simulink model "TestHz"  (R2020b)
settings: Solver=FixedStepDiscrete  StartTime=0.0  StopTime=inf  FixedStep=Ts  RelTol=1e-3
values from neighbouring files (symbols this model uses):
  g = 9.81    [equpoint.m]    (also in plotAMS.m; plotAMS2.m)
  J = diag([0.0056 0.0056 0.0104])    [equpoint.m]
  m = 0.7    [equpoint.m]    (also in plotAMS.m = 0.752; plotAMS2.m = 0.752)
  M = ([ 1          1          1         1 ... (first row only)    [allocation.m]    (also in equpoint.m; plotAMS.m; plotAMS2.m)
undefined symbols (not defined in the file or in its folder): B, MY_ATT_P, MY_ATT_P_YAW, MY_POS_P, MY_RATE_P, MY_RATE_P_YAW, MY_SAT_AD, MY_TAU_P_A, MY_TAU_P_A_YAW, MY_TAU_P_P, MY_TAU_P_P_YAW, MY_VEL_P, T00, Tf, Tmotorbar, Ts
libraries: discretizing x10, pixhawk_slib_uORB_RW x6, pixhawk_slib_sensors_actuators x5, pixhawk_slib_misc_utils x1, simulink x1, sharedtransform x1, pid_lib x1
(part 1 of 2)
settings Model: Creator=kcx06  LastModifiedBy=kcx06
settings SolverCC: PositivePriorityOrder=on  AutoInsertRateTranBlk=on
settings DataIOCC: SaveOutput=off  DSMLogging=off  SaveTime=off  ReturnWorkspaceOutputs=off
settings OptimizationCC: DefaultParameterBehavior=Inlined  EnhancedBackFolding=on  PassReuseOutputArgsAs=Individual arguments  ZeroExternalMemoryAtStartup=off  ZeroInternalMemoryAtStartup=off  MaxStackSize=64  OptimizeBlockOrder=speed  DifferentSizesBufferReuse=on  OptimizationCustomize=off  EfficientTunableParamExpr=on
settings DebuggingCC: ParameterTunabilityLossMsg=error
settings HardwareCC: ProdBitPerPointer=32  ProdBitPerSizeT=32  ProdBitPerPtrDiffT=32  ProdLargestAtomicInteger=Long  ProdLargestAtomicFloat=Double  ProdWordSize=32  ProdHWDeviceType=ARM Compatible->ARM Cortex
settings SFSimCC: MATLABDynamicMemAlloc=off
settings RTWCC: Description=Embedded Coder  SystemTargetFile=ert.tlc  HardwareBoard=Pixhawk PX4  TLCOptions="-aInlineSetEventsForThisBaseRateFcn=TLC_FALSE -aSuppressMultiTaskScheduler=TLC_FALSE  -aRateBasedStepFcn=0"  TemplateMakefile=ert_default_tmf  GenerateReport=on  CustomSource=px4_simulink_app_params.c  Toolchain=Pixhawk Toolchain  BuildConfiguration=Faster Runs  LaunchReport=on
settings CodeAppCC: ForceParamTrailComments=on  IgnoreCustomStorageClasses=off  OperatorAnnotations=on  SimulinkDataObjDesc=on  SFDataObjDesc=on  InsertBlockDesc=on
settings ERTTargetCC: SupportComplex=off  SupportContinuousTime=on  InlinedParameterPlacement=NonHierarchical  ERTCustomFileTemplate=px4_codertarget_file_process.tlc

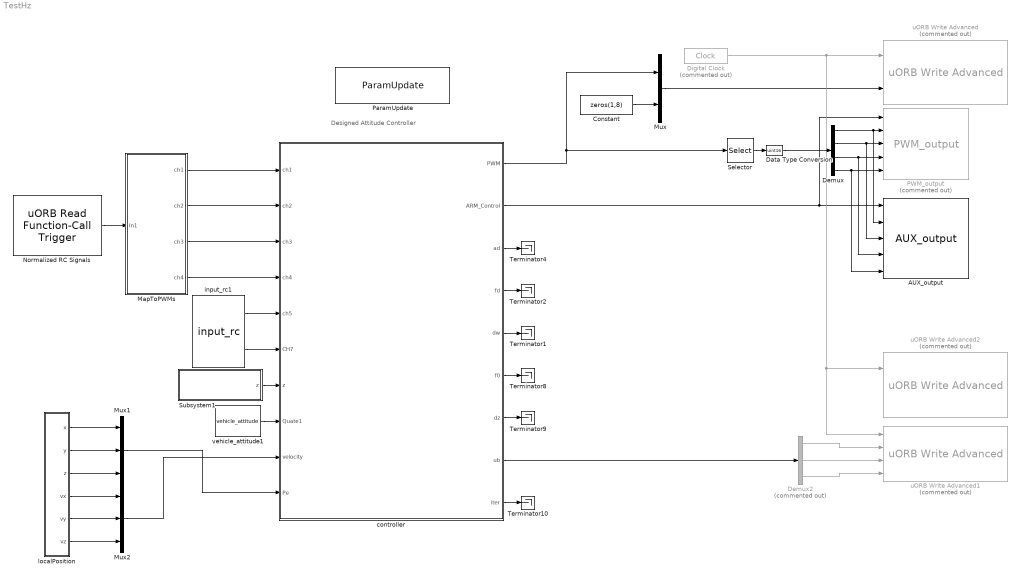
== system TestHz ==
  note: Designed Attitude Controller
  AUX_output : pixhawk_slib_sensors_actuators/AUX_output  Description=|  pwm_rate=400Hz  show_aux1=on  show_aux4=on  show_aux2=on  show_aux5=off  show_aux3=on  show_aux6=off
      | This block allows the user to send the appropriate PWM signals out to the PX4 AUX outputs.  
      | These are usually connected to the ESCs which control the motor speeds. 
      | In order for the flight control to arm (enable) the output from the software side, the ARM Output input must be held high (boolean TRUE).  
      | Only then will the PWM values be sent out the PX4 hardware ports.  
      | This is usually a function of the RC Tx in combination with other flight modes programmed in the Simulink model by the user.  
      | The block has 8 available ports (data type uint16) which can be selectively chosen.  
      | These correspond to the 6 PWM (optional on 5/6) output ports on the px4fmu hardware. 
      | 
      | You *must* ensure that the line: “fmu mode_pwm” appears in your rc.txt file or manually run this from a Nuttx terminal *before* you start the px4_simulink_app module.  
      | Also – note: the FMU only has to be ARMED for the AUX pins to work – the Hardware safety switch is only for the IO.  
      | The switch’s blink code tells you what is armed.  You have to ARM both the Hardware switch and Software block in order to get the PWM output to work, but only the Software block for the AUX outputs.
      settings: SourceProductName=Pixhawk Target Blocks
  Constant : Constant  Value=zeros(1,8)  OutDataTypeStr=single
  Data Type Conversion : DataTypeConversion  OutDataTypeStr=uint16
  Demux : Demux
  Demux2 : Demux  Commented=on  Outputs=3
  Digital Clock : DigitalClock  Commented=on  SampleTime=Ts
  MapToPWMs : Subsystem
  Mux : Mux  Inputs=2
  Mux1 : Mux  Inputs=3
  Mux2 : Mux  Inputs=3
  Normalized RC Signals : pixhawk_slib_uORB_RW/uORB Read Function-Call Trigger  uORB_Topic_str='manual_control_setpoint'  BusObjVar=Bus: manual_control_setpoint_SL  uORB_Interval=1  AsyncOutput=off  Fcn_call_select=Generate Function Call Signal  TaskName='Task1'  Poll_timeout=100  Ts=Ts
      settings: SourceProductName=Pixhawk Target Blocks
  PWM_output : pixhawk_slib_sensors_actuators/PWM_output  Description=|  Commented=on  pub_outputs=on  pwm_rate=400Hz  show_pwm1=on  show_pwm5=off  show_pwm2=on  show_pwm6=off  show_pwm3=on  show_pwm7=off  show_pwm4=on  show_pwm8=off
      | This block allows the user to send the appropriate PWM signals out to the PX4 outputs.  
      | These are usually connected to the ESCs which control the motor speeds. 
      | In order for the flight control to arm (enable) the output from the software side, the ARM Output input must be held high (boolean TRUE).  
      | Only then will the PWM values be sent out the PX4 hardware ports.  
      | This is usually a function of the RC Tx in combination with other flight modes programmed in the Simulink model by the user.  
      | The block has 8 available ports (data type uint16) which can be selectively chosen.  
      | These correspond to the 8 PWM output ports on the px4fmu hardware.
      settings: SourceProductName=Pixhawk Target Blocks
  ParamUpdate : pixhawk_slib_misc_utils/ParamUpdate  Description=|  Unformatted_StrSet=0  TLC_StrSet=0  NumParams=0  Ts=0
      | ParamUpdate Block
      | 
      | Use this block at your top-level of your model to insert a "parameter update" function in the generated code.
      settings: SourceProductName=Pixhawk Target Blocks
  Selector : Selector  IndexMode=Zero-based  InputPortWidth=8  IndexOptions=Index vector (dialog)  Indices=[0 1 2 3]  OutputSizes=1
  Subsystem1 : Subsystem
  Terminator{1..2,4,8..10} (6 alike) : Terminator
  controller : Subsystem
  input_rc1 : pixhawk_slib_sensors_actuators/input_rc  Description=|  sampletime=1/50  channel1=off  channel2=off  channel3=off  channel4=off  channel5=on  channel6=on  channel7=off  channel8=off  channel9=off  channel10=off  channel11=off  channel12=off  channel13=off  channel14=off  channel15=off  channel16=off  channel17=off  channel18=off  ch_count=off  rssi=off  rc_failsafe=off  rc_lost=off  rc_inputsource=off
      | RC Input Block
      | 
      | This block provides user input control to the model.
      | It uses the input_rc uORB topic.
      | 
      | The user has the ability to choose which channels are available as outputs from this block and also some optional outputs. These include 
      | Channels 1 through 18
      | double data type indicating the PWM value from the controller 
      | measured pulse widths for each of the supported channels 
      | Channel Count 
      | uint32 data type of the number of channels which are detector by the PX4 
      | RC Failsafe 
      | boolean data types indicating that the RC Tx is sending the FailSafe signal (if equipped and properly setup) 
      | explicit failsafe flag: true on TX failure or TX out of range , false otherwise. 
      | Only the true state is reliable, as there are some (PPM) receivers on the market going into failsafe without telling us explicitly. 
      | RC Input Source 
      | Enumeration data type indicating which source the RC input is from. 
      | Valid values are found in the ENUM file: RC_INPUT_SOURCE_ENUM.m 
      |           Enumeration members for class 'RC_INPUT_SOURCE_ENUM':
      |           RCINPUT_SOURCE_UNKNOWN         (0)
      |           RCINPUT_SOURCE_PX4FMU_PPM      (1)
      |           RCINPUT_SOURCE_PX4IO_PPM       (2)
      |           RCINPUT_SOURCE_PX4IO_SPEKTRUM  (3)
      |           RCINPUT_SOURCE_PX4IO_SBUS      (4)
      |           RCINPUT_SOURCE_PX4IO_ST24      (5)
      |           RCINPUT_SOURCE_MAVLINK         (6)
      |           RCINPUT_SOURCE_QURT            (7)
      |           RCINPUT_SOURCE_PX4FMU_SPEKTRUM (8)
      |           RCINPUT_SOURCE_PX4FMU_SBUS     (9)
      |           RCINPUT_SOURCE_PX4FMU_ST24     (10)
      |           RCINPUT_SOURCE_PX4FMU_SUMD     (11)
      |           RCINPUT_SOURCE_PX4FMU_DSM      (12)
      |           RCINPUT_SOURCE_PX4IO_SUMD      (13)
      | 
      | RSSI - Receive signal strength index 
      | receive signal strength indicator (RSSI): < 0: Undefined, 0: no signal, 255: full reception 
      | RC Lost Connection 
      | boolean data type indicating RC receiver connection status 
      | True, if no frame has arrived in the expected time, false otherwise. 
      | True usally means that the receiver has been disconnected, but can also indicate a radio link loss on "stupid" systems. 
      | Will remain false, if a RX with failsafe option continues to transmit frames after a link loss. 
      |   
      | Sample Model: px4demo_input_rc.slx
      settings: SourceProductName=Pixhawk Target Blocks
  "localPosition " : Subsystem
  uORB Write Advanced : pixhawk_slib_uORB_RW/uORB Write Advanced  Commented=on  Ts=0  uORB_AdvtQueue=on  uORB_FieldEnabledArr="0  0  0  1  0  0  0  0  0  0  0"  uORB_Topic_str=0  uORB_Struct_DT="[1  1  1  1  1]"  BlockInputCount=5  uORB_StructParams="[\"voltage_v\",\"voltage_filtered_v\",\"current_a\",\"current_filtered_a\",\"remaining\"]"  uORB_PortSizes="[1  1  1  1]"  MsgSizeOf=0  MW_update=true
      settings: SourceProductName=Pixhawk Target Blocks
  uORB Write Advanced1 : pixhawk_slib_uORB_RW/uORB Write Advanced  Commented=on  Ts=0  uORB_AdvtQueue=on  uORB_FieldEnabledArr="0  0  0  1  0  0  0  0  0  0  0"  uORB_Topic_str=0  uORB_Struct_DT="[1  1  1  1  1]"  BlockInputCount=5  uORB_StructParams="[\"voltage_v\",\"voltage_filtered_v\",\"current_a\",\"current_filtered_a\",\"remaining\"]"  uORB_PortSizes="[1  1  1  1]"  MsgSizeOf=0  MW_update=true
      settings: SourceProductName=Pixhawk Target Blocks
  uORB Write Advanced2 : pixhawk_slib_uORB_RW/uORB Write Advanced  Commented=on  Ts=0  uORB_AdvtQueue=on  uORB_FieldEnabledArr="0  0  0  1  0  0  0  0  0  0  0"  uORB_Topic_str=0  uORB_Struct_DT="[1  1  1  1  1]"  BlockInputCount=5  uORB_StructParams="[\"voltage_v\",\"voltage_filtered_v\",\"current_a\",\"current_filtered_a\",\"remaining\"]"  uORB_PortSizes="[1  1  1  1]"  MsgSizeOf=0  MW_update=true
      settings: SourceProductName=Pixhawk Target Blocks
  vehicle_attitude1 : pixhawk_slib_sensors_actuators/vehicle_attitude  sampletime=Ts  show_r=off  show_p=off  show_y=off  show_q=on  show_ts=off
      settings: SourceProductName=Pixhawk Target Blocks
  wires:
  controller/3(ad) -> Terminator4/1
  controller/1(PWM) -> Selector/1, Mux/1
  controller/2(ARM_Control) -> AUX_output/1, PWM_output/1
  MapToPWMs/4(ch4) -> controller/4(ch4)
  Constant/1 -> Mux/2
  controller/5(dw) -> Terminator1/1
  "localPosition "/5(vy) -> Mux2/2
  MapToPWMs/1(ch1) -> controller/1(ch1)
  input_rc1/1 -> controller/5(ch5)
  Mux1/1 -> controller/10(Pe)
  "localPosition "/3(z) -> Mux1/3
  Mux2/1 -> controller/9(velocity)
  controller/4(fd) -> Terminator2/1
  "localPosition "/4(vx) -> Mux2/1
  MapToPWMs/3(ch3) -> controller/3(ch3)
  "localPosition "/2(y) -> Mux1/2
  Normalized RC Signals/1 -> MapToPWMs/1(In1)
  Mux/1 -> uORB Write Advanced/2
  "localPosition "/1(x) -> Mux1/1
  MapToPWMs/2(ch2) -> controller/2(ch2)
  Digital Clock/1 -> uORB Write Advanced1/1, uORB Write Advanced2/1, uORB Write Advanced/1
  controller/8(ub) -> Demux2/1
  "localPosition "/6(vz) -> Mux2/3
  input_rc1/2 -> controller/6(CH7)
  controller/6(f0) -> Terminator8/1
  controller/7(dz) -> Terminator9/1
  controller/9(iter) -> Terminator10/1
  vehicle_attitude1/1 -> controller/8(Quate1)
  Subsystem1/1(z) -> controller/7(z)
  Selector/1 -> Data Type Conversion/1
  Demux/1 -> AUX_output/2, PWM_output/2
  Demux/2 -> PWM_output/3, AUX_output/3
  Demux/3 -> AUX_output/4, PWM_output/4
  Demux/4 -> AUX_output/5, PWM_output/5
  Data Type Conversion/1 -> Demux/1
  Demux2/3 -> uORB Write Advanced1/4
  Demux2/1 -> uORB Write Advanced1/2
  Demux2/2 -> uORB Write Advanced1/3

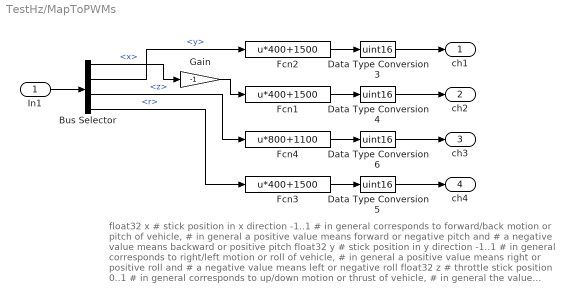
== system TestHz/MapToPWMs ==
  note: float32 x			 # stick position in x direction -1..1
      | 				 # in general corresponds to forward/back motion or pitch of vehicle,
      | 				 # in general a positive value means forward or negative pitch and
      | 				 # a negative value means backward or positive pitch
      | float32 y			 # stick position in y direction -1..1
      | 				 # in general corresponds to right/left motion or roll of vehicle,
      | 				 # in general a positive value means right or positive roll and
      | 				 # a negative value means left or negative roll
      | float32 z			 # throttle stick position 0..1
      | 				 # in general corresponds to up/down motion or thrust of vehicle,
      | 				 # in general the value corresponds to the demanded throttle by the user,
      | 				 # if the input is used for setting the setpoint of a vertical position
      | 				 # controller any value > 0.5 means up and any value < 0.5 means down
      | float32 r			 # yaw stick/twist position, -1..1
      | 				 # in general corresponds to the righthand rotation around the vertical
      | 				 # (downwards) axis of the vehicle
  In1 : Inport
  Bus Selector : BusSelector  OutputSignals=x,y,z,r
  Data Type Conversion{3..6} (4 alike) : DataTypeConversion  OutDataTypeStr=uint16
  Fcn1 : Fcn  Expr=u*400+1500
  Fcn2 : Fcn  Expr=u*400+1500
  Fcn3 : Fcn  Expr=u*400+1500
  Fcn4 : Fcn  Expr=u*800+1100
  Gain : Gain  Gain=-1
  ch1 : Outport  VectorParamsAs1DForOutWhenUnconnected=off
  ch2 : Outport  Port=2  VectorParamsAs1DForOutWhenUnconnected=off
  ch3 : Outport  Port=3  VectorParamsAs1DForOutWhenUnconnected=off
  ch4 : Outport  Port=4  VectorParamsAs1DForOutWhenUnconnected=off
  wires:
  Bus Selector/2 -> Fcn2/1  "<y>"
  Fcn2/1 -> Data Type Conversion3/1
  Bus Selector/1 -> Gain/1  "<x>"
  In1/1 -> Bus Selector/1
  Bus Selector/3 -> Fcn4/1  "<z>"
  Fcn1/1 -> Data Type Conversion4/1
  Bus Selector/4 -> Fcn3/1  "<r>"
  Data Type Conversion4/1 -> ch2/1
  Data Type Conversion5/1 -> ch4/1
  Data Type Conversion6/1 -> ch3/1
  Fcn4/1 -> Data Type Conversion6/1
  Fcn3/1 -> Data Type Conversion5/1
  Data Type Conversion3/1 -> ch1/1
  Gain/1 -> Fcn1/1

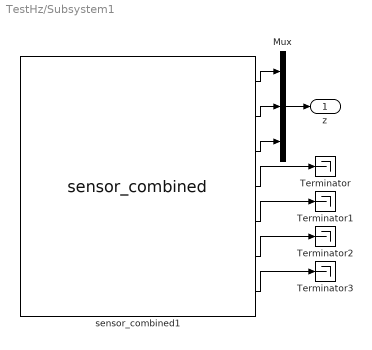
== system TestHz/Subsystem1 ==
  Mux : Mux  Inputs=3
  Terminator{,1..3} (4 alike) : Terminator
  sensor_combined1 : pixhawk_slib_sensors_actuators/sensor_combined  Description=|  sampletime=Ts  show_mag=off  show_acc=off  show_gyro=on  show_baro=off  show_ts=on
      | Sensor Combined Block
      | 
      | This block enables access to the various sensors available on the px4fmu-v2 hardware.  
      | The user can use these signals in the Simulink control model.  
      | The sample time needs to be provided in the mask dialog.  
      | Optional output ports can also be selected.  
      | Refer to the sample model: px4demo_attitude_control.slx
      | 
      | Signal definitions: 
      | Magnetometer (x,y,z) - single values – Magnetic field in NED body frame, in Gauss 
      | Accelerometer (x,y,z) - single values – Acceleration in NED body frame, in m/s^2 
      | Gyroscope (p,q,r) - single values – Angular velocity in radians per second 
      | Barometer (Altitude) - single value – Barometric pressure, already temperature compensated (millibars) 
      | RunTime (timestamp) - double value – Timestamp in microseconds since boot, from gyro 
      |   
      | The sensor_combined block needs to have the px4io service running on the PX4 hardware in order to get valid signal values.
      settings: SourceProductName=Pixhawk Target Blocks
  z : Outport
  wires:
  Mux/1 -> z/1
  sensor_combined1/1 -> Mux/1
  sensor_combined1/2 -> Mux/2
  sensor_combined1/3 -> Mux/3
  sensor_combined1/4 -> Terminator/1
  sensor_combined1/5 -> Terminator1/1
  sensor_combined1/6 -> Terminator2/1
  sensor_combined1/7 -> Terminator3/1

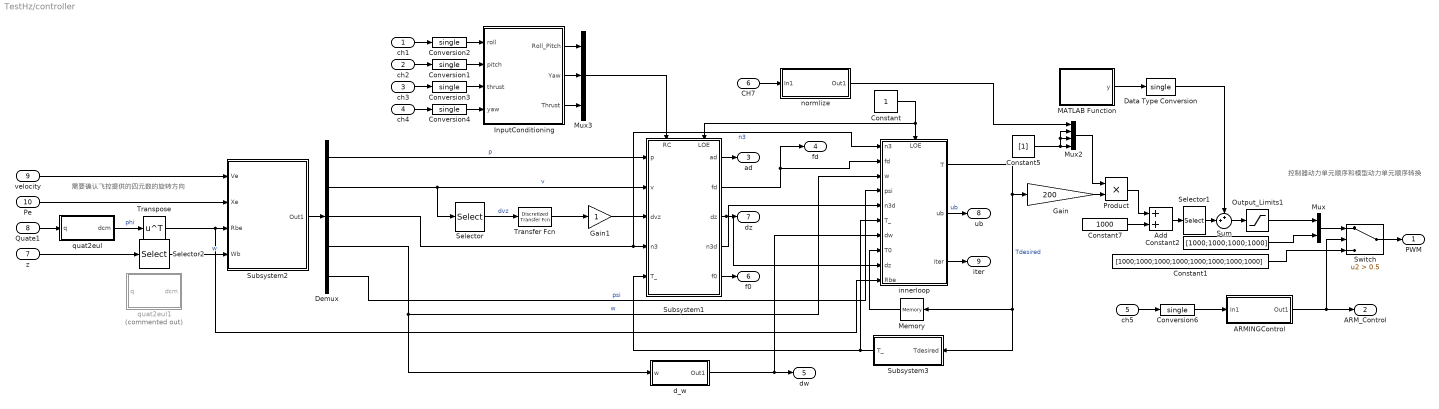
== system TestHz/controller ==
  note: 需要确认飞控提供的四元数的旋转方向
  note: 控制器动力单元顺序和模型动力单元顺序转换
  ch1 : Inport  OutDataTypeStr=uint16  PortDimensions=1
  ch2 : Inport  Port=2  OutDataTypeStr=uint16  PortDimensions=1
  ch3 : Inport  Port=3  OutDataTypeStr=uint16  PortDimensions=1
  ch4 : Inport  Port=4  OutDataTypeStr=uint16  PortDimensions=1
  ch5 : Inport  Port=5  OutDataTypeStr=uint16  PortDimensions=1  Interpolate=off
  CH7 : Inport  Port=6
  z : Inport  Port=7
  Quate1 : Inport  Port=8
  velocity : Inport  Port=9
  Pe : Inport  Port=10
  ARMINGControl : Subsystem
  Add : Sum
  Constant : Constant  OutDataTypeStr=single
  Constant1 : Constant  Value=[1000;1000;1000;1000;1000;1000;1000;1000]  OutDataTypeStr=single
  Constant2 : Constant  Value=[1000;1000;1000;1000]  OutDataTypeStr=single
  Constant5 : Constant  Value=[1]  OutDataTypeStr=single
  Constant7 : Constant  Value=1000  OutDataTypeStr=single
  Conversion{1..4,6} (5 alike) : DataTypeConversion  OutDataTypeStr=single
  Data Type Conversion : DataTypeConversion  OutDataTypeStr=single
  Demux : Demux  Outputs=[3 3 3 3 1]
  Gain : Gain  Gain=200
  Gain1 : Gain
  InputConditioning : Subsystem
  MATLAB Function : MATLAB Function  TreatAsAtomicUnit=on
  Memory : Memory  InitialCondition=T00
  Mux : Mux  Inputs=2
  Mux2 : Mux
  Mux3 : Mux  Inputs=3
  Output_Limits1 : Saturate  UpperLimit=2000  LowerLimit=1000
  Product : Product
  Selector : Selector  IndexMode=Zero-based  InputPortWidth=3  IndexOptions=Index vector (dialog)  Indices=[2]  OutputSizes=1
  Selector1 : Selector  IndexMode=Zero-based  InputPortWidth=4  IndexOptions=Index vector (dialog)  Indices=[0 2 3 1]  OutputSizes=1
  Selector2 : Selector  IndexMode=Zero-based  InputPortWidth=3  IndexOptions=Index vector (dialog)  Indices=[0 1 2]  OutputSizes=1
  Subsystem1 : Subsystem
      settings: PortSchema="{\"entries\":[{\"content\":{\"sides\":[{\"content\":{\"connectorIds\":[\"In1\",\"In2\",\"In3\",\"In4\",\"In5\"]},\"type\":\"ConnectorPlacement.EquallySpacedRectSide\",\"uuid\":\"59983f3e-2daf-41bd-bc3f-074c85f4b2eb\"},{\"content\":{\"connectorIds\":[\"Out1\",\"Out2\",\"Out3\",\"Out4\",\"Out5\"],\"side\":\"RIGHT\"},\"type\":\"ConnectorPlacement.EquallySpacedRectSide\",\"uuid\":\"6ee11e40-7870-4737-b9e6-fd7c25119100\"},{\"content\":{\"connectorIds\":[\"In6\",\"In7\"],\"side\":\"TOP\"},\"type\":\"ConnectorPlacement.EquallySpacedRectSide\",\"uuid\":\"847e9a02-4621-4cf8-a675-1479afa28be0\"}]},\"type\":\"ConnectorPlacement.EquallySpacedConnector\",\"uuid\":\"28981c41-e87e-4da3-ac2d-04a56d75ff2b\"}],\"packageUris\":[\"http://schema.mathworks.com/mf0/Connector/19700101\"],\"version\":\"1.0\"}"
  Subsystem2 : Subsystem
  Subsystem3 : Subsystem
  Sum : Sum  Inputs=++|
  Switch : Switch  Criteria=u2 > Threshold  Threshold=0.5
  Transfer Fcn : discretizing/Discretized Transfer Fcn  Numerator=[1 0]  Denominator=[Tf 1]  AbsTol=auto  SampleTime=Ts  method=zoh  Wc=1
      settings: SourceProductBaseCode=SL
  Transpose : Math  Operator=transpose  SaturateOnIntegerOverflow=on
  d_w : Subsystem
  innerloop : Subsystem
      settings: PortSchema="{\"entries\":[{\"content\":{\"sides\":[{\"content\":{\"connectorIds\":[\"In1\",\"In2\",\"In3\",\"In4\",\"In5\",\"In6\",\"In7\",\"In8\",\"In9\",\"In10\"]},\"type\":\"ConnectorPlacement.EquallySpacedRectSide\",\"uuid\":\"43c6e1bd-c98b-47b4-98da-f51fdffff433\"},{\"content\":{\"connectorIds\":[\"Out1\",\"Out2\",\"Out3\"],\"side\":\"RIGHT\"},\"type\":\"ConnectorPlacement.EquallySpacedRectSide\",\"uuid\":\"ac1c9532-9168-4bf4-8fed-08d3fdc16453\"},{\"content\":{\"connectorIds\":[\"In11\"],\"side\":\"TOP\"},\"type\":\"ConnectorPlacement.EquallySpacedRectSide\",\"uuid\":\"32774b13-030c-47c6-b846-fc6c0ce2dd6f\"}]},\"type\":\"ConnectorPlacement.EquallySpacedConnector\",\"uuid\":\"dd62421a-d766-429a-a161-5a0f77c5a7ba\"}],\"packageUris\":[\"http://schema.mathworks.com/mf0/Connector/19700101\"],\"version\":\"1.0\"}"
  normlize : Subsystem
  quat2eul : MATLAB Function  TreatAsAtomicUnit=on
  quat2eul1 : MATLAB Function  Commented=on  TreatAsAtomicUnit=on
  PWM : Outport  PortDimensions=8  VectorParamsAs1DForOutWhenUnconnected=off
  ARM_Control : Outport  Port=2  PortDimensions=1  VectorParamsAs1DForOutWhenUnconnected=off
  ad : Outport  Port=3
  fd : Outport  Port=4
  dw : Outport  Port=5
  f0 : Outport  Port=6
  dz : Outport  Port=7
  ub : Outport  Port=8
  iter : Outport  Port=9
  wires:
  ARMINGControl/1(Out1) -> Switch/2, ARM_Control/1
  Conversion4/1 -> InputConditioning/4(yaw)
  Output_Limits1/1 -> Mux/1
  ch4/1 -> Conversion4/1
  ch2/1 -> Conversion1/1
  ch5/1 -> Conversion6/1
  Conversion1/1 -> InputConditioning/2(pitch)
  Conversion6/1 -> ARMINGControl/1(In1)
  Conversion2/1 -> InputConditioning/1(roll)
  ch1/1 -> Conversion2/1
  ch3/1 -> Conversion3/1
  Constant2/1 -> Mux/2
  Mux/1 -> Switch/1
  Constant1/1 -> Switch/3
  innerloop/1(T) -> Subsystem3/1(Tdesired), Memory/1, Gain/1  "Tdesired"
  Demux/5 -> innerloop/4(psi)  "psi"
  Memory/1 -> innerloop/8(T0)
  Selector/1 -> Transfer Fcn/1  "dvz"
  Demux/4 -> d_w/1(w), innerloop/3(w)  "w"
  Demux/2 -> Selector/1, Subsystem1/2(v)  "v"
  Selector1/1 -> Sum/2
  Constant7/1 -> Add/2
  Gain/1 -> Product/2
  Add/1 -> Selector1/1
  innerloop/2(ub) -> ub/1  "ub"
  Subsystem2/1(Out1) -> Demux/1
  Selector2/1 -> Subsystem2/4(Wb)  "w"
  velocity/1 -> Subsystem2/1(Ve)
  Pe/1 -> Subsystem2/2(Xe)
  Quate1/1 -> quat2eul/1(q)
  Conversion3/1 -> InputConditioning/3(thrust)
  d_w/1(Out1) -> innerloop/7(dw), dw/1
  quat2eul/1(dcm) -> Transpose/1  "phi"
  Subsystem1/2(fd) -> fd/1, innerloop/2(fd)
  Demux/1 -> Subsystem1/1(p)  "p"
  Transfer Fcn/1 -> Gain1/1
  Subsystem1/1(ad) -> ad/1
  Subsystem1/3(dz) -> innerloop/9(dz), dz/1
  Subsystem1/4(n3d) -> innerloop/5(n3d)
  Subsystem1/5(f0) -> f0/1
  Subsystem3/1(T_) -> innerloop/6(T_), Subsystem1/5(T_)
  CH7/1 -> normlize/1(In1)
  Constant/1 -> Subsystem1/7(LOE), innerloop/11(LOE)
  Mux2/1 -> Product/1
  Product/1 -> Add/1
  Gain1/1 -> Subsystem1/3(dvz)
  Constant5/1 -> Mux2/3, Mux2/2, Mux2/4
  innerloop/3(iter) -> iter/1
  Transpose/1 -> innerloop/10(Rbe), Subsystem2/3(Rbe)
  Demux/3 -> innerloop/1(n3), Subsystem1/4(n3)  "n3"
  InputConditioning/1(Roll_Pitch) -> Mux3/1
  InputConditioning/2(Yaw) -> Mux3/2
  InputConditioning/3(Thrust) -> Mux3/3
  z/1 -> Selector2/1
  Mux3/1 -> Subsystem1/6(RC)
  Switch/1 -> PWM/1
  normlize/1(Out1) -> Mux2/1
  Sum/1 -> Output_Limits1/1
  MATLAB Function/1(y) -> Data Type Conversion/1
  Data Type Conversion/1 -> Sum/1

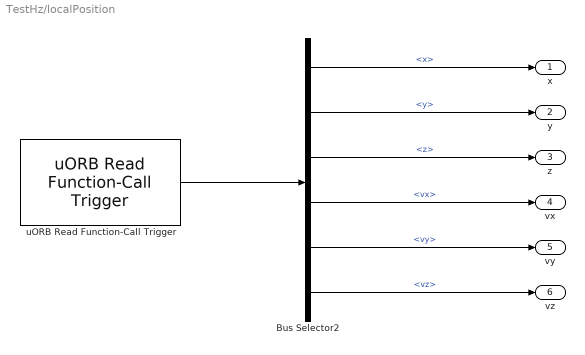
== system TestHz/localPosition  ==
  Bus Selector2 : BusSelector  OutputSignals=x,y,z,vx,vy,vz
  uORB Read Function-Call Trigger : pixhawk_slib_uORB_RW/uORB Read Function-Call Trigger  uORB_Topic_str='vehicle_local_position'  BusObjVar=Bus: vehicle_local_position_SL  uORB_Interval=1  AsyncOutput=off  Fcn_call_select=Generate Function Call Signal  TaskName='Task1'  Poll_timeout=100  Ts=Ts
      settings: SourceProductName=Pixhawk Target Blocks
  x : Outport  VectorParamsAs1DForOutWhenUnconnected=off
  y : Outport  Port=2  VectorParamsAs1DForOutWhenUnconnected=off
  z : Outport  Port=3  VectorParamsAs1DForOutWhenUnconnected=off
  vx : Outport  Port=4  VectorParamsAs1DForOutWhenUnconnected=off
  vy : Outport  Port=5  VectorParamsAs1DForOutWhenUnconnected=off
  vz : Outport  Port=6  VectorParamsAs1DForOutWhenUnconnected=off
  wires:
  uORB Read Function-Call Trigger/1 -> Bus Selector2/1
  Bus Selector2/6 -> vz/1  "<vz>"
  Bus Selector2/5 -> vy/1  "<vy>"
  Bus Selector2/4 -> vx/1  "<vx>"
  Bus Selector2/1 -> x/1  "<x>"
  Bus Selector2/2 -> y/1  "<y>"
  Bus Selector2/3 -> z/1  "<z>"

== system TestHz/controller/ARMINGControl ==
  In1 : Inport
  Compare To Constant3 : simulink/Logic and Bit Operations/Compare To Constant  relop=>=  const=uint16(1500)  OutDataTypeStr=boolean
  Out1 : Outport  VectorParamsAs1DForOutWhenUnconnected=off
  wires:
  Compare To Constant3/1 -> Out1/1
  In1/1 -> Compare To Constant3/1

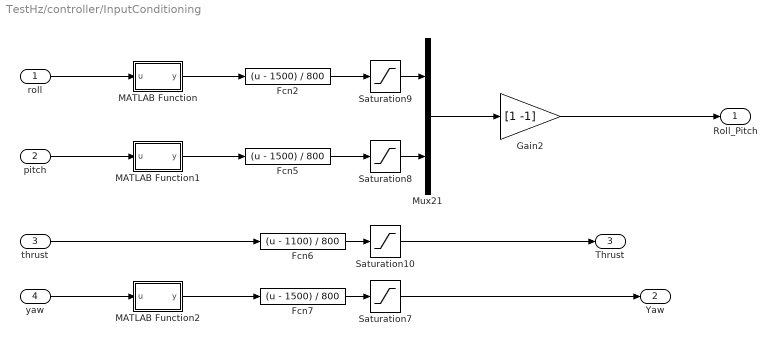
== system TestHz/controller/InputConditioning ==
  roll : Inport
  pitch : Inport  Port=2
  thrust : Inport  Port=3
  yaw : Inport  Port=4
  Fcn2 : Fcn  Expr=(u - 1500) / 800
  Fcn5 : Fcn  Expr=(u - 1500) / 800
  Fcn6 : Fcn  Expr=(u - 1100) / 800
  Fcn7 : Fcn  Expr=(u - 1500) / 800
  Gain2 : Gain  Gain=[1 -1]  OutDataTypeStr=Inherit: Inherit via back propagation
  MATLAB Function : MATLAB Function  TreatAsAtomicUnit=on
  MATLAB Function1 : MATLAB Function  TreatAsAtomicUnit=on
  MATLAB Function2 : MATLAB Function  TreatAsAtomicUnit=on
  Mux21 : Mux  Inputs=2
  Saturation10 : Saturate  UpperLimit=1  LowerLimit=0
  Saturation7 : Saturate  UpperLimit=1  LowerLimit=-1
  Saturation8 : Saturate  UpperLimit=1  LowerLimit=-1
  Saturation9 : Saturate  UpperLimit=1  LowerLimit=-1
  Roll_Pitch : Outport  VectorParamsAs1DForOutWhenUnconnected=off
  Yaw : Outport  Port=2  VectorParamsAs1DForOutWhenUnconnected=off
  Thrust : Outport  Port=3  VectorParamsAs1DForOutWhenUnconnected=off
  wires:
  Saturation10/1 -> Thrust/1
  Saturation7/1 -> Yaw/1
  Gain2/1 -> Roll_Pitch/1
  Mux21/1 -> Gain2/1
  Saturation8/1 -> Mux21/2
  Fcn6/1 -> Saturation10/1
  Fcn2/1 -> Saturation9/1
  Fcn5/1 -> Saturation8/1
  Saturation9/1 -> Mux21/1
  Fcn7/1 -> Saturation7/1
  pitch/1 -> MATLAB Function1/1(u)
  MATLAB Function2/1(y) -> Fcn7/1
  thrust/1 -> Fcn6/1
  roll/1 -> MATLAB Function/1(u)
  MATLAB Function1/1(y) -> Fcn5/1
  MATLAB Function/1(y) -> Fcn2/1
  yaw/1 -> MATLAB Function2/1(u)

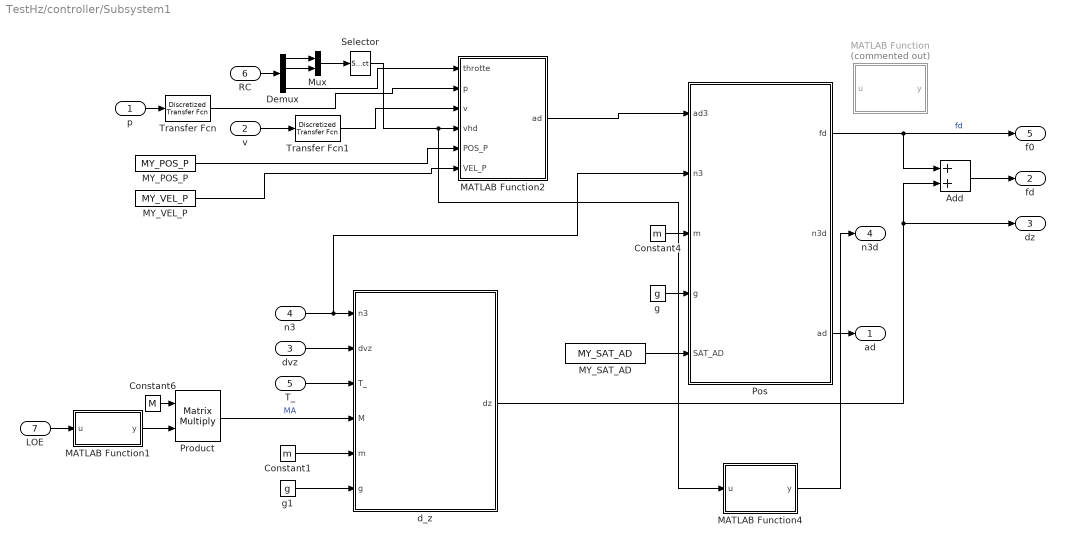
== system TestHz/controller/Subsystem1 ==
  p : Inport
  v : Inport  Port=2
  dvz : Inport  Port=3
  n3 : Inport  Port=4
  T_ : Inport  Port=5
  RC : Inport  Port=6
  LOE : Inport  Port=7
  Add : Sum
  Constant1 : Constant  Value=m  OutDataTypeStr=single
  Constant4 : Constant  Value=m  OutDataTypeStr=single
  Constant6 : Constant  Value=M  OutDataTypeStr=single
  Demux : Demux
  MATLAB Function : MATLAB Function  Commented=on  TreatAsAtomicUnit=on
  MATLAB Function1 : MATLAB Function  TreatAsAtomicUnit=on
  MATLAB Function2 : MATLAB Function  TreatAsAtomicUnit=on
  MATLAB Function4 : MATLAB Function  TreatAsAtomicUnit=on
  MY_POS_P : Constant  Value=MY_POS_P
  MY_SAT_AD : Constant  Value=MY_SAT_AD
      settings: AttributesFormatString=|
      | 0.13
      | Default
  MY_VEL_P : Constant  Value=MY_VEL_P
  Mux : Mux  Inputs=2
  Pos : MATLAB Function  TreatAsAtomicUnit=on
  Product : Product  Multiplication=Matrix(*)
  Selector : Selector  IndexMode=Zero-based  InputPortWidth=2  IndexOptions=Index vector (dialog)  Indices=[1 0]  OutputSizes=1
  Transfer Fcn : discretizing/Discretized Transfer Fcn  Numerator=[1 ]  Denominator=[Tf 1]  AbsTol=auto  SampleTime=Ts  method=zoh  Wc=1
      settings: SourceProductBaseCode=SL
  Transfer Fcn1 : discretizing/Discretized Transfer Fcn  Numerator=[1 ]  Denominator=[Tf 1]  AbsTol=auto  SampleTime=Ts  method=zoh  Wc=1
      settings: SourceProductBaseCode=SL
  d_z : MATLAB Function  TreatAsAtomicUnit=on
  g : Constant  Value=g  OutDataTypeStr=single
  g1 : Constant  Value=g  OutDataTypeStr=single
  ad : Outport
  fd : Outport  Port=2
  dz : Outport  Port=3
  n3d : Outport  Port=4
  f0 : Outport  Port=5
  wires:
  Pos/3(ad) -> ad/1
  dvz/1 -> d_z/2(dvz)
  Pos/1(fd) -> f0/1, Add/1  "fd"
  p/1 -> Transfer Fcn/1
  T_/1 -> d_z/3(T_)
  v/1 -> Transfer Fcn1/1
  Constant4/1 -> Pos/3(m)
  g/1 -> Pos/4(g)
  Constant1/1 -> d_z/5(m)
  g1/1 -> d_z/6(g)
  Add/1 -> fd/1
  d_z/1(dz) -> dz/1, Add/2
  Transfer Fcn/1 -> MATLAB Function2/2(p)
  n3/1 -> Pos/2(n3), d_z/1(n3)
  MATLAB Function1/1(y) -> Product/2
  LOE/1 -> MATLAB Function1/1(u)
  Constant6/1 -> Product/1
  Product/1 -> d_z/4(M)  "MA"
  RC/1 -> Demux/1
  Demux/4 -> MATLAB Function2/1(throtte)
  MATLAB Function2/1(ad) -> Pos/1(ad3)
  Transfer Fcn1/1 -> MATLAB Function2/3(v)
  Demux/1 -> Mux/1
  Demux/2 -> Mux/2
  Mux/1 -> Selector/1
  Selector/1 -> MATLAB Function4/1(u), MATLAB Function2/4(vhd)
  MY_POS_P/1 -> MATLAB Function2/5(POS_P)
  MY_VEL_P/1 -> MATLAB Function2/6(VEL_P)
  MY_SAT_AD/1 -> Pos/5(SAT_AD)
  MATLAB Function4/1(y) -> n3d/1

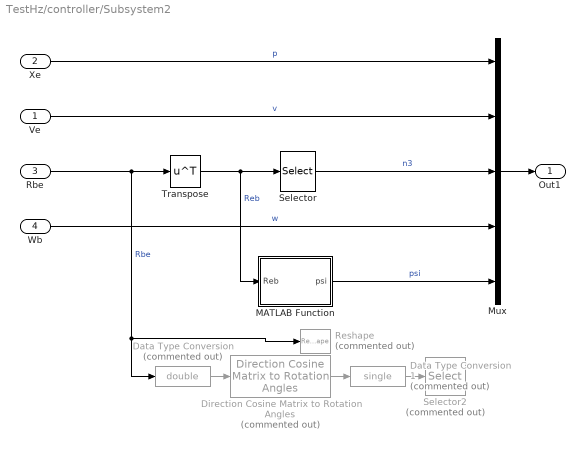
== system TestHz/controller/Subsystem2 ==
  Ve : Inport
  Xe : Inport  Port=2
  Rbe : Inport  Port=3
  Wb : Inport  Port=4
  Data Type Conversion : DataTypeConversion  Commented=on  OutDataTypeStr=double
  Data Type Conversion1 : DataTypeConversion  Commented=on  OutDataTypeStr=single
  Direction Cosine Matrix to Rotation Angles : sharedtransform/Direction Cosine Matrix to Rotation Angles  Commented=on  rotationOrder=ZYX  aMode=aMode  action=None  tolerance=eps(2)
      settings: SourceProductBaseCode=AE,PW,MT,UV,VE,VP
  MATLAB Function : MATLAB Function  TreatAsAtomicUnit=on
  Mux : Mux  Inputs=[3 3 3 3 1]
  Reshape : Reshape  Commented=on
  Selector : Selector  NumberOfDimensions=2  IndexMode=Zero-based  InputPortWidth=3  IndexOptions=Select all,Index vector (dialog)  Indices=[1 3],2  OutputSizes=1,1
  Selector2 : Selector  Commented=on  InputPortWidth=3  IndexOptions=Index vector (dialog)  Indices=[3 2 1]  OutputSizes=1
  Transpose : Math  Operator=transpose  SaturateOnIntegerOverflow=on
  Out1 : Outport
  wires:
  Xe/1 -> Mux/1  "p"
  Ve/1 -> Mux/2  "v"
  Rbe/1 -> Reshape/1, Data Type Conversion/1, Transpose/1  "Rbe"
  Transpose/1 -> MATLAB Function/1(Reb), Selector/1  "Reb"
  Selector/1 -> Mux/3  "n3"
  Mux/1 -> Out1/1
  Wb/1 -> Mux/4  "w"
  MATLAB Function/1(psi) -> Mux/5  "psi"
  Direction Cosine Matrix to Rotation Angles/1 -> Data Type Conversion1/1
  Data Type Conversion/1 -> Direction Cosine Matrix to Rotation Angles/1
  Data Type Conversion1/1 -> Selector2/1

== system TestHz/controller/Subsystem3 ==
  Tdesired : Inport
  Transfer Fcn10 : discretizing/Discretized Transfer Fcn  Numerator=[1]  Denominator=[Tmotorbar 1]  AbsTol=auto  SampleTime=Ts  method=zoh  Wc=1
      settings: SourceProductBaseCode=SL
  Transfer Fcn9 : discretizing/Discretized Transfer Fcn  Numerator=[1]  Denominator=[Tf 1]  AbsTol=auto  SampleTime=Ts  method=zoh  Wc=1
      settings: SourceProductBaseCode=SL
  T_ : Outport
  wires:
  Transfer Fcn10/1 -> T_/1
  Tdesired/1 -> Transfer Fcn9/1
  Transfer Fcn9/1 -> Transfer Fcn10/1

== system TestHz/controller/d_w ==
  w : Inport
  Transfer Fcn4 : discretizing/Discretized Transfer Fcn  Numerator=[1 0]  Denominator=[Tf 1]  AbsTol=auto  SampleTime=Ts  method=zoh  Wc=1
      settings: SourceProductBaseCode=SL
  Out1 : Outport
  wires:
  w/1 -> Transfer Fcn4/1
  Transfer Fcn4/1 -> Out1/1

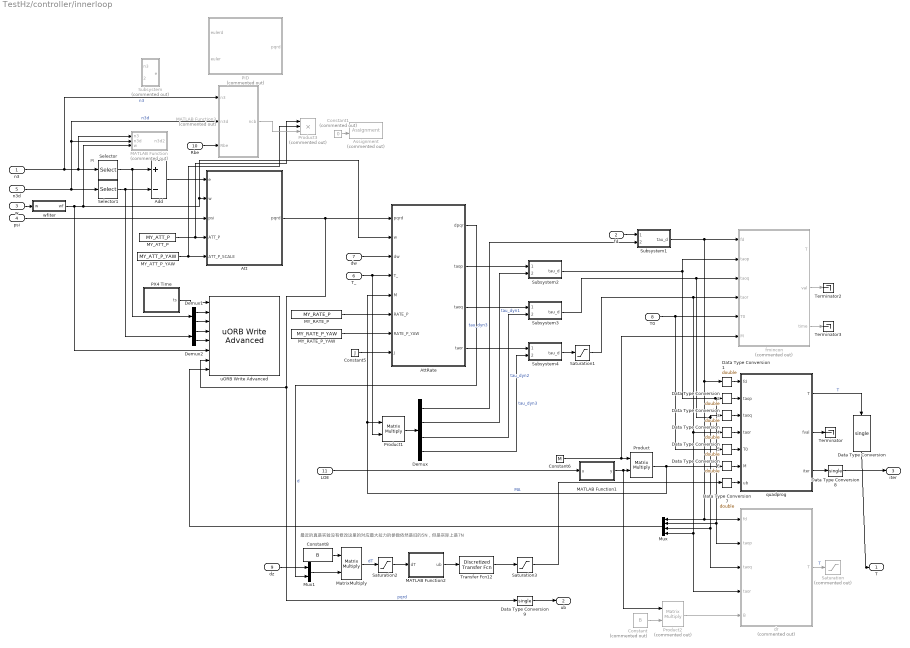
== system TestHz/controller/innerloop ==
  note: PI
  note: 最近的真是实验没有修改这里的对应最大拉力的参数依然是旧的5N，但是实际上是7N
  n3 : Inport
  fd : Inport  Port=2
  w : Inport  Port=3
  psi : Inport  Port=4
  n3d : Inport  Port=5
  T_ : Inport  Port=6
  dw : Inport  Port=7
  T0 : Inport  Port=8
  dz : Inport  Port=9
  Rbe : Inport  Port=10
  LOE : Inport  Port=11
  Add : Sum  Inputs=+-
  Assignment : Assignment  Commented=on  DiagnosticForDimensions=Warning  IndexOptions=Index vector (dialog)  Indices=3  OutputSizes=1
  Att : MATLAB Function  TreatAsAtomicUnit=on
  AttRate : MATLAB Function  TreatAsAtomicUnit=on
  Constant : Constant  Commented=on  Value=B  OutDataTypeStr=single
  Constant1 : Constant  Commented=on  Value=0  OutDataTypeStr=single
  Constant5 : Constant  Value=J  OutDataTypeStr=single
  Constant6 : Constant  Value=M  OutDataTypeStr=single
  Constant8 : Constant  Value=B
  Data Type Conversion : DataTypeConversion  OutDataTypeStr=single
  Data Type Conversion{1..7} (7 alike) : DataTypeConversion  OutDataTypeStr=double
  Data Type Conversion8 : DataTypeConversion  OutDataTypeStr=single
  Data Type Conversion9 : DataTypeConversion  OutDataTypeStr=single
  Demux : Demux
  Demux1 : Demux  Outputs=2
  Demux2 : Demux  Outputs=2
  MATLAB Function : MATLAB Function  Commented=on  TreatAsAtomicUnit=on
  MATLAB Function1 : MATLAB Function  TreatAsAtomicUnit=on
  MATLAB Function2 : MATLAB Function  TreatAsAtomicUnit=on
  MATLAB Function3 : MATLAB Function  Commented=on  TreatAsAtomicUnit=on
  MY_ATT_P : Constant  Value=MY_ATT_P
  MY_ATT_P_YAW : Constant  Value=MY_ATT_P_YAW
  MY_RATE_P : Constant  Value=MY_RATE_P
  MY_RATE_P_YAW : Constant  Value=MY_RATE_P_YAW
  MatrixMultiply : Product  Multiplication=Matrix(*)
  Mux : Mux
  Mux1 : Mux  Inputs=2
  PID : MATLAB Function  Commented=on  TreatAsAtomicUnit=on
  PX4 Time : MATLAB Function  TreatAsAtomicUnit=on
  Product : Product  Multiplication=Matrix(*)
  Product1 : Product  Multiplication=Matrix(*)
  Product2 : Product  Commented=on  Multiplication=Matrix(*)
  Product3 : Product  Commented=on  Inputs=3
  Saturation : Saturate  Commented=on  UpperLimit=[3 3 3 3]  LowerLimit=[0 0 0 0]  OutDataTypeStr=single
  Saturation1 : Saturate  UpperLimit=0.075  LowerLimit=-0.075
  Saturation2 : Saturate  UpperLimit=5  LowerLimit=-5
  Saturation3 : Saturate  UpperLimit=5  LowerLimit=0
  Selector : Selector  IndexMode=Zero-based  InputPortWidth=3  IndexOptions=Index vector (dialog)  Indices=[0 1]  OutputSizes=1
  Selector1 : Selector  IndexMode=Zero-based  InputPortWidth=3  IndexOptions=Index vector (dialog)  Indices=[0 1]  OutputSizes=1
  Subsystem : Subsystem  Commented=on
  Subsystem1 : Subsystem
  Subsystem2 : Subsystem
  Subsystem3 : Subsystem
  Subsystem4 : Subsystem
  Terminator : Terminator
  Terminator2 : Terminator
  Terminator3 : Terminator
  Transfer Fcn12 : discretizing/Discretized Transfer Fcn  Numerator=[1]  Denominator="[1.7  1]"  AbsTol=auto  SampleTime=Ts  method=zoh  Wc=40
      link override Discrete Transfer Fcn: InitialStates=[5;5;5;5]
      settings: SourceProductBaseCode=SL
  dr : MATLAB Function  Commented=on  TreatAsAtomicUnit=on
  fmincon : MATLAB Function  Commented=on  TreatAsAtomicUnit=on
  quadprog : MATLAB Function  TreatAsAtomicUnit=on
  uORB Write Advanced : pixhawk_slib_uORB_RW/uORB Write Advanced  Ts=0  uORB_AdvtQueue=on  uORB_FieldEnabledArr="0  0  0  1  0  0  0  0  0  0  0"  uORB_Topic_str=0  uORB_Struct_DT="[1  1  1  1  1]"  BlockInputCount=5  uORB_StructParams="[\"voltage_v\",\"voltage_filtered_v\",\"current_a\",\"current_filtered_a\",\"remaining\"]"  uORB_PortSizes="[1  1  1  1]"  MsgSizeOf=0  MW_update=true
      settings: SourceProductName=Pixhawk Target Blocks
  wfiter : Subsystem
  T : Outport  PortDimensions=4
  ub : Outport  Port=2
  iter : Outport  Port=3
  wires:
  dw/1 -> AttRate/3(dw)
  AttRate/1(dpqr) -> Mux1/2  "d"
  T0/1 -> fmincon/5(T0), Data Type Conversion5/1
  T_/1 -> Product1/2, AttRate/4(T_)
  Constant5/1 -> AttRate/8(J)
  Constant6/1 -> fmincon/6(M), Product/1
  quadprog/2(fval) -> Terminator/1
  dr/1(T) -> Saturation/1  "T"
  fmincon/2(val) -> Terminator2/1
  fmincon/3(time) -> Terminator3/1
  Product2/1 -> dr/5(B)
  psi/1 -> Att/3(psi)
  w/1 -> wfiter/1(w)
  wfiter/1(wf) -> uORB Write Advanced/6, MATLAB Function/3(w), AttRate/2(w), Att/2(w)
  quadprog/1(T) -> Data Type Conversion/1  "T"
  Data Type Conversion1/1 -> quadprog/1(fd)
  Data Type Conversion2/1 -> quadprog/2(taop)
  Data Type Conversion3/1 -> quadprog/3(taoq)
  Data Type Conversion4/1 -> quadprog/4(taor)
  Data Type Conversion5/1 -> quadprog/5(T0)
  Data Type Conversion6/1 -> quadprog/6(M)
  Data Type Conversion7/1 -> quadprog/7(ub)
  Subsystem2/1(tau_d) -> fmincon/2(taop), Mux/2, dr/2(taop), Data Type Conversion2/1
  Subsystem3/1(tau_d) -> Mux/3, dr/3(taoq), Data Type Conversion3/1, fmincon/3(taoq)
  Subsystem4/1(tau_d) -> Saturation1/1
  Subsystem1/1(tau_d) -> Mux/1, dr/1(fd), Data Type Conversion1/1, fmincon/1(fd)
  quadprog/3(iter) -> Data Type Conversion8/1
  Data Type Conversion8/1 -> iter/1
  Demux/1 -> Subsystem1/2(tau_dyn)  "tau_dyn3"
  fd/1 -> Subsystem1/1(tau_dynd)
  AttRate/2(taop) -> Subsystem2/1(tau_dynd)
  Demux/2 -> Subsystem2/2(tau_dyn)  "tau_dyn1"
  AttRate/3(taoq) -> Subsystem3/1(tau_dynd)
  Demux/3 -> Subsystem3/2(tau_dyn)  "tau_dyn2"
  AttRate/4(taor) -> Subsystem4/1(tau_dynd)
  Demux/4 -> Subsystem4/2(tau_dyn)  "tau_dyn3"
  Saturation1/1 -> Mux/4, dr/4(taor), Data Type Conversion4/1, fmincon/4(taor)
  LOE/1 -> MATLAB Function1/1(u)
  Product/1 -> Product1/1, AttRate/5(M), Data Type Conversion6/1  "MA"
  n3/1 -> MATLAB Function3/1(n3), Selector/1, MATLAB Function/1(n3)  "n3"
  Product1/1 -> Demux/1
  Att/1(pqrd) -> AttRate/1(pqrd), Data Type Conversion9/1, uORB Write Advanced/7  "pqrd"
  Constant/1 -> Product2/2
  MATLAB Function1/1(y) -> Product2/1, Product/2
  Data Type Conversion/1 -> T/1
  MY_RATE_P/1 -> AttRate/6(RATE_P)
  MY_RATE_P_YAW/1 -> AttRate/7(RATE_P_YAW)
  MY_ATT_P/1 -> Att/4(ATT_P), Product3/1
  MY_ATT_P_YAW/1 -> Product3/2, Att/5(ATT_P_SCALE)
  n3d/1 -> MATLAB Function/2(n3d), MATLAB Function3/2(n3d), Selector1/1  "n3d"
  MATLAB Function2/1(ub) -> Transfer Fcn12/1
  Constant8/1 -> MatrixMultiply/1
  Mux1/1 -> MatrixMultiply/2
  dz/1 -> Mux1/1
  Saturation2/1 -> MATLAB Function2/1(dT)
  MatrixMultiply/1 -> Saturation2/1  "dT"
  Transfer Fcn12/1 -> Saturation3/1
  Saturation3/1 -> Data Type Conversion7/1
  Add/1 -> Att/1(e)
  Data Type Conversion9/1 -> ub/1
  Rbe/1 -> MATLAB Function3/3(Rbe)
  MATLAB Function3/1(ncb) -> Product3/3
  Constant1/1 -> Assignment/2
  Demux2/2 -> uORB Write Advanced/5
  Demux1/2 -> uORB Write Advanced/3
  PX4 Time/1(ts) -> uORB Write Advanced/1
  Demux1/1 -> uORB Write Advanced/2
  Selector1/1 -> Add/2, Demux2/1
  Selector/1 -> Add/1, Demux1/1
  Demux2/1 -> uORB Write Advanced/4
  Mux/1 -> uORB Write Advanced/8

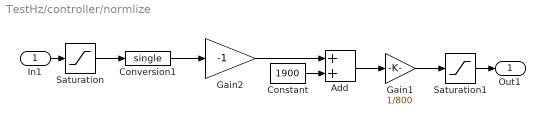
== system TestHz/controller/normlize ==
  In1 : Inport
  Add : Sum
  Constant : Constant  Value=1900  OutDataTypeStr=single
  Conversion1 : DataTypeConversion  OutDataTypeStr=single
  Gain1 : Gain  Gain=1/800
  Gain2 : Gain  Gain=-1
  Saturation : Saturate  UpperLimit=1900  LowerLimit=1100
  Saturation1 : Saturate  UpperLimit=1  LowerLimit=0
  Out1 : Outport
  wires:
  Saturation/1 -> Conversion1/1
  Gain2/1 -> Add/1
  Gain1/1 -> Saturation1/1
  Add/1 -> Gain1/1
  In1/1 -> Saturation/1
  Constant/1 -> Add/2
  Conversion1/1 -> Gain2/1
  Saturation1/1 -> Out1/1

== system TestHz/controller/innerloop/Subsystem ==
  n3 : Inport
  n3d : Inport  Port=2
  Add : Sum  Inputs=+-
  PID Controller : pid_lib/PID Controller  Commented=on  Controller=PI  Form=Parallel  TimeDomain=Discrete-time  UseExternalTs=off  SampleTime=-1  IntegratorMethod=Forward Euler  FilterMethod=Forward Euler  ControllerParametersSource=internal  P=0.8  I=0.05  D=0.02  UseFilter=on  N=100  TunerSelectOption=Transfer Function Based (PID Tuner App)  InitialConditionSource=internal  InitialConditionForIntegrator=0  InitialConditionForFilter=0  DifferentiatorICPrevScaledInput=0  ExternalReset=none  TrackingMode=off  Kt=1  LimitOutput=off  SatLimitsSource=internal  UpperSaturationLimit=0.3  LowerSaturationLimit=-0.3  LinearizeAsGain=on  AntiWindupMode=clamping  Kb=1  POutMin=[]  POutMax=[]  IOutMin=[]  IOutMax=[]  DOutMin=[]  DOutMax=[]  NOutMin=[]  NOutMax=[]  SumOutMin=[]  SumOutMax=[]  SaturationOutMin=[]  SaturationOutMax=[]  PParamMin=[]  PParamMax=[]  IParamMin=[]  IParamMax=[]  DParamMin=[]  DParamMax=[]  NParamMin=[]  NParamMax=[]  KbParamMin=[]  KbParamMax=[]  KtParamMin=[]  KtParamMax=[]  KbOutMin=[]  KbOutMax=[]  KtOutMin=[]  KtOutMax=[]  IntegratorOutMin=[]  IntegratorOutMax=[]  FilterOutMin=[]  FilterOutMax=[]  SumI1OutMin=[]  SumI1OutMax=[]  SumI2OutMin=[]  SumI2OutMax=[]  SumI3OutMin=[]  SumI3OutMax=[]  SumI4OutMin=[]  SumI4OutMax=[]  SumDOutMin=[]  SumDOutMax=[]  DifferentiatorOutMin=[]  DifferentiatorOutMax=[]  FilterDiffOutCoefMin=[]  FilterDiffOutCoefMax=[]  ReciprocalOutMin=[]  ReciprocalOutMax=[]  SumDenOutMin=[]  SumDenOutMax=[]  SumNumOutMin=[]  SumNumOutMax=[]  DivideOutMin=[]  DivideOutMax=[]  UdiffTsProdOutMin=[]  UdiffTsProdOutMax=[]  NTsProdOutMin=[]  NTsProdOutMax=[]  UintegralTsProdOutMin=[]  UintegralTsProdOutMax=[]  UngainTsProdOutMin=[]  UngainTsProdOutMax=[]  IntegratorContinuousStateAttributes=''  IntegratorStateMustResolveToSignalObject=off  IntegratorRTWStateStorageClass=Auto  FilterContinuousStateAttributes=''  FilterStateMustResolveToSignalObject=off  FilterRTWStateStorageClass=Auto  ParallelPVariant=InternalParameters  IdealPVariant=Disabled  IVariant=InternalParameters  DVariant=Disabled  IntegratorVariant=Discrete  SatVariant=Disabled  AWVariant=Passthrough  PCopyVariant=Disabled  TRVariant=Disabled  FdbkBlocksVariant=Forward  IdealPFdbkVariant=Disabled  SatFdbkVariant=Disabled  DerivativeFilterVariant=Disabled  NVariant=Disabled  NCopyVariant=Disabled_SignalSpec  FilterICVariant=Disabled  IntegratorICVariant=InternalICs  ExternalResetVariant=Disabled  TRSumVariant=Passthrough  SumFdbkVariant=Disabled  SumVariant=Sum_PI  TsampFilterVariant=InternalTs  TsampNgainVariant=Passthrough  TsampIntegralVariant=Passthrough  ExternalSaturationOutDataTypeStr=Inherit: Same as second input
  Selector : Selector  IndexMode=Zero-based  InputPortWidth=3  IndexOptions=Index vector (dialog)  Indices=[0 1]  OutputSizes=1
  Selector1 : Selector  IndexMode=Zero-based  InputPortWidth=3  IndexOptions=Index vector (dialog)  Indices=[0 1]  OutputSizes=1
  e : Outport
  wires:
  n3/1 -> Selector/1
  n3d/1 -> Selector1/1
  Selector/1 -> Add/1
  Selector1/1 -> Add/2
  Add/1 -> e/1

== system TestHz/controller/innerloop/Subsystem1 ==
  tau_dynd : Inport
  tau_dyn : Inport  Port=2
  Gain7 : Gain
  Sum1 : Sum  Inputs=|++
  Sum4 : Sum  Inputs=|+-
  tau_d : Outport
  wires:
  tau_dynd/1 -> Sum4/1  "omega"
  Gain7/1 -> Sum1/1
  Sum4/1 -> Gain7/1
  Sum1/1 -> tau_d/1
  tau_dyn/1 -> Sum1/2, Sum4/2

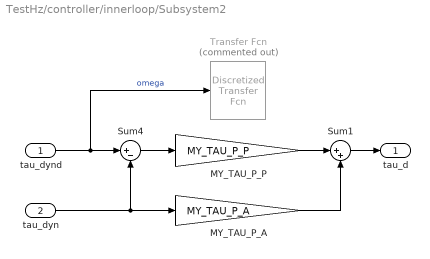
== system TestHz/controller/innerloop/Subsystem2 ==
  tau_dynd : Inport
  tau_dyn : Inport  Port=2
  MY_TAU_P_A : Gain  Gain=MY_TAU_P_A
  MY_TAU_P_P : Gain  Gain=MY_TAU_P_P
  Sum1 : Sum  Inputs=|++
  Sum4 : Sum  Inputs=|+-
  Transfer Fcn : discretizing/Discretized Transfer Fcn  Commented=on  Numerator=[0.005 0]  Denominator=[Tf 1]  AbsTol=auto  SampleTime=Ts  method=zoh  Wc=1
      settings: SourceProductBaseCode=SL
  tau_d : Outport
  wires:
  tau_dyn/1 -> Sum4/2, MY_TAU_P_A/1
  Sum1/1 -> tau_d/1
  Sum4/1 -> MY_TAU_P_P/1
  tau_dynd/1 -> Transfer Fcn/1, Sum4/1  "omega"
  MY_TAU_P_A/1 -> Sum1/2
  MY_TAU_P_P/1 -> Sum1/1

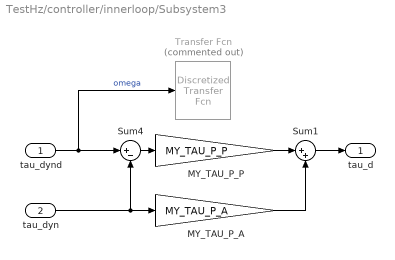
== system TestHz/controller/innerloop/Subsystem3 ==
  tau_dynd : Inport
  tau_dyn : Inport  Port=2
  MY_TAU_P_A : Gain  Gain=MY_TAU_P_A
  MY_TAU_P_P : Gain  Gain=MY_TAU_P_P
  Sum1 : Sum  Inputs=|++
  Sum4 : Sum  Inputs=|+-
  Transfer Fcn : discretizing/Discretized Transfer Fcn  Commented=on  Numerator=[0.005 0]  Denominator=[Tf 1]  AbsTol=auto  SampleTime=Ts  method=zoh  Wc=1
      settings: SourceProductBaseCode=SL
  tau_d : Outport
  wires:
  tau_dynd/1 -> Transfer Fcn/1, Sum4/1  "omega"
  Sum4/1 -> MY_TAU_P_P/1
  Sum1/1 -> tau_d/1
  tau_dyn/1 -> Sum4/2, MY_TAU_P_A/1
  MY_TAU_P_A/1 -> Sum1/2
  MY_TAU_P_P/1 -> Sum1/1

== system TestHz/controller/innerloop/Subsystem4 ==
  tau_dynd : Inport
  tau_dyn : Inport  Port=2
  MY_TAU_P_A_YAW : Gain  Gain=MY_TAU_P_A_YAW
  MY_TAU_P_P_YAW : Gain  Gain=MY_TAU_P_P_YAW
  Sum1 : Sum  Inputs=|++
  Sum4 : Sum  Inputs=|+-
  tau_d : Outport
  wires:
  tau_dyn/1 -> MY_TAU_P_A_YAW/1, Sum4/2
  Sum1/1 -> tau_d/1
  Sum4/1 -> MY_TAU_P_P_YAW/1
  MY_TAU_P_P_YAW/1 -> Sum1/1
  tau_dynd/1 -> Sum4/1  "omega"
  MY_TAU_P_A_YAW/1 -> Sum1/2

== system TestHz/controller/innerloop/wfiter ==
  w : Inport
  Transfer Fcn4 : discretizing/Discretized Transfer Fcn  Numerator=[1]  Denominator=[Tf 1]  AbsTol=auto  SampleTime=Ts  method=zoh  Wc=1
      settings: SourceProductBaseCode=SL
  wf : Outport
  wires:
  Transfer Fcn4/1 -> wf/1
  w/1 -> Transfer Fcn4/1

== matlab function TestHz/controller/Subsystem1/MATLAB Function ==
  data: u input; y output
function y = fcn(u)
if u<0.9
y = single(0);
else
y = single(1);
end

== matlab function TestHz/controller/Subsystem1/MATLAB Function1 ==
  data: u input; y output
function y = fcn(u)
y=diag([u,1,1,1]);

== matlab function TestHz/controller/quat2eul1 ==
  data: q input single; dcm output single
function dcm  = quat2eul(q)
% Conversion from Quaternion to Euler angles based on the PX4 Firmware
% v1.6.5 release.
% 
% Quaternion -> DCM -> Euler Angles
% INPUT:
%   q: Quaternion vector of the format: (a + bi + cj + dk)
% OUTPUT:
%   [phi,theta,psi]: Euler angles in radians.
% 
 if norm(q)~=0
    a = q(1);
    b = q(2);
    c = q(3);
    d = q(4);

    aSq = a*a;
    bSq = b*b;
    cSq = c*c;
    dSq = d*d;

    d_pi2 = pi/2;

    % quaternion_to_dcm
    dcm00 = aSq + bSq - cSq - dSq;
    dcm01 = 2*(b*c - a*d);
    dcm02 = 2*(a*c + b*d);
    dcm10 = 2*(b*c + a*d);
    dcm11 = aSq - bSq + cSq - dSq;
    dcm12 = 2*(c*d - a*b);
    dcm20 = 2*(b*d - a*c);
    dcm21 = 2*(a*b + c*d);
    dcm22 = aSq - bSq - cSq + dSq;
    dcm=[dcm00 dcm01 dcm02;
              dcm10 dcm11 dcm12;
              dcm20 dcm21  dcm22];
 else
     dcm = single(eye(3,3));
 end
    % dcm_to_euler

== matlab function TestHz/controller/innerloop/MATLAB Function ==
  data: n3 input; n3d2 output; n3d input; w input
function n3d2 = fcn(n3, n3d, w)
if abs(w(3))>pi
    % costheta   = dot(n3, n3d);
    costhetaXY = dot([n3(1:2);0], [n3d(1:2);0])/(norm([n3(1:2);0])*norm([n3d(1:2);0]));
    % sintheta   = cross(n3, n3d);
    sinthetaXY = cross([n3(1:2);0], [n3d(1:2);0])/(norm([n3(1:2);0])*norm([n3d(1:2);0]));

%     if sinthetaXY(3) > 0  
        %俯视下顺时针，与1号电机停止后机体旋转方向相反，不符合陀螺进动方向      
    %% s1 没有测试（预计没有明显改善）   
    %     n3d = [-n3d(1)/1; -n3d(2)/1; n3d(3)];
    %% s2 位置超调略大
    %     n3d = [single(0); single(0); single(1.0)];
    %% s3 位置超调过大
    %     n3d = [-n3(1)/3; -n3(2)/3; n3(3)];
    %     n3d = n3d/norm(n3d); 
%     end


    %% s4
    % if costhetaXY <0.9397  %只考虑夹角大小不管转向是否符合陀螺进动方向,大于20°满足
    %     n3d = [single(0); single(0); single(1.0)];
    % end

    %% s5
    if costhetaXY <0.8660 && sinthetaXY(3) > 0 %考虑夹角大小和是否符合陀螺进动方向大于20°满足
        n3d = [single(0); single(0); single(1.0)];
    end

    %% s6
    % if costheta <0.9397  %只考虑夹角大小不管转向是否符合陀螺进动方向,大于20°满足
    %     n3d = [single(0); single(0); single(1.0)];
    % end

    %% s7
    % if costheta <0.9397 && sinthetaXY(3) > 0 %考虑夹角大小和是否符合陀螺进动方向大于20°满足
    %     n3d = [single(0); single(0); single(1.0)];
    % end
end
n3d2 = n3d;

== matlab function TestHz/controller/innerloop/PID ==
  data: eulerd input; euler input; pqrd output
function pqrd  = fcn(eulerd, euler)
k1 = 3;
pqd = k1 * [eulerd(1)-euler(1);eulerd(2)-euler(2)];
pqrd = [pqd;0];

== matlab function TestHz/controller/innerloop/MATLAB Function3 ==
  data: n3 input; ncb output; n3d input; Rbe input
function ncb = fcn(n3, n3d, Rbe)
nc = cross(n3, n3d);
ncb  = Rbe*nc;

== matlab function TestHz/controller/Subsystem1/MATLAB Function4 ==
  data: u input; y output
function y = fcn(u)
y = [-u/4; 1]/norm([-u/4; 1]);

== matlab function TestHz/controller/innerloop/PX4 Time ==
  data: ts output
function ts  = fcn
% coder.cinclude('drivers/drv_hrt.h');
persistent count
if isempty(count)
    count = 0;
end

hrt = 0;
if coder.target('Rtw')
    hrt = coder.ceval('hrt_absolute_time');
else
    hrt = count;
end
ts = hrt;% us

count = count + 1;

== matlab function TestHz/controller/MATLAB Function ==
  data: y output
function y = fcn()
persistent count
if isempty(count)
 count =0;
end
if count == 0
    y = [1000;1000;1000;1000];
    count = 1;
else
    y = [0;0;0;0];
    count = 0;
end

== matlab function TestHz/controller/innerloop/AttRate ==
  data: pqrd input; w input; dw input; T_ input; M input; RATE_P input; RATE_P_YAW input; J input; dpqr output size=3; taop output; taoq output; taor output
function [dpqr, taop, taoq, taor] = fcn(pqrd, w, dw, T_, M, RATE_P, RATE_P_YAW, J)
pqd = pqrd(1:2);
rd    = pqrd(3);
%% 角速率控制器计算

k2 = RATE_P;
k2_scaled = k2*RATE_P_YAW;

% kr = 0.001;
% dp =  M(2,:)*T_ - J(1,1)*dw(1) - kr*abs(w(1))*w(1) + w(2)*w(3)*(J(2,2)-J(3,3));
% dq =  M(3,:)*T_ - J(2,2)*dw(2) - kr*abs(w(2))*w(2) + w(3)*w(1)*(J(3,3)-J(1,1));
% dr  =  M(4,:)*T_ - J(3,3)*dw(3) - kr*abs(w(3))*w(3) + w(1)*w(2)*(J(1,1)-J(2,2));
dp = M(2,:)*T_ -J(1,1)*dw(1);
dq = M(3,:)*T_ -J(2,2)*dw(2);
dr  = M(4,:)*T_ -J(3,3)*dw(3);

% taop =            J(1,1)*k2*(pqd(1)-w(1)) + kr*abs(w(1))*w(1) - w(2)*w(3)*(J(2,2)-J(3,3))+dp;
% taoq =            J(2,2)*k2*(pqd(2)-w(2)) + kr*abs(w(2))*w(2) - w(3)*w(1)*(J(3,3)-J(1,1))+dq;
% taor  = mysatsingle(J(3,3)*k2_scaled*(rd-w(3)) + kr*abs(w(3))*w(3) - w(1)*w(2)*(J(1,1)-J(2,2))+dr,10.0);
taop =           J(1,1)*k2*(pqd(1)-w(1))+1.0*dp;
taoq =           J(2,2)*k2*(pqd(2)-w(2))+1.0*dq;
taor  = mysatsingle(J(3,3)*k2_scaled*(rd-w(3))+1.0*dr,1.0);

dpqr = [dp; dq; dr];

== matlab function TestHz/controller/innerloop/dr ==
  data: fd input single size=1; taop input single size=1; taoq input single size=1; taor input single size=1; T output single size=4; B input single size=[4,4]
function T  = fcn(fd, taop, taoq, taor, B)
%% 求解
vd = [fd; taop; taoq; taor];

T1 = B(1,:)*vd;
T2 = B(2,:)*vd;
T3 = B(3,:)*vd;
T4 = B(4,:)*vd;
T = [T1; T2; T3; T4];
% T=min(max(B*vd,[single(0);single(0);single(0);single(0)]),[single(3); single(3); single(3); single(3)]);

== matlab function TestHz/controller/innerloop/fmincon ==
  data: fd input; taop input; taoq input; taor input; T output; T0 input; M input; val output; time output
function [T,val,time] = fcn(fd, taop, taoq, taor, T0, M)
%% 求解
w1= 1;
w2 =20;
w3= 20;
w4= 0.00;
myfun2 = @(x)(w1*(M(1,:)*x-fd)^2+w2*(M(2,:)*x-taop)^2+w3*(M(3,:)*x-taoq)^2+w4*(M(4,:)*x-taor)^2);

lb  = [0 0 0 0]';
ub  = [3 3 3 3]';

options = optimoptions(@fmincon,'Algorithm','sqp','MaxIterations',10);
% tic
[T,val] = fmincon(myfun2,T0,[],[],[],[],lb,ub,[],options);
% ff = toc;
time =0;

== matlab function TestHz/controller/innerloop/quadprog ==
  data: fd input double; taop input double; taoq input double; taor input double; T output double; T0 input double; M input double; fval output double; ub input double; iter output
function [T,fval, iter] = fcn(fd, taop, taoq, taor, T0, M, ub)
%% 求解
vd = [fd; taop; taoq; taor];
W=diag([1 20 20 0.01]);
H = M'*W*M;
f = -(vd'*W*M)';
% Td = B*vd;
lb  = [0 0 0 0]';
% ub  = [12 12 12 12]';
% if (max(B*vd)>3)||(min(B*vd)<0)
    options = optimoptions(@quadprog,'Algorithm','active-set','MaxIterations',10);

    [T,fval,~,output] = quadprog(H, f, [], [], [], [], lb, ub, T0, options);
     iter = output.iterations;
% else
%     T = B*vd;
%     fval = 0;
% end
